simulink model "forme_canoniche"  (R2021b)
settings: Solver=ode3  StartTime=0.0  StopTime=2  FixedStep=Ts  RelTol=1e-3
values from neighbouring files (symbols this model uses):
  a = a(2:end)    [script.m]
  b = 2    [script.m]
  R = 1    [script.m]
settings Model: Creator=antony  LastModifiedBy=antony

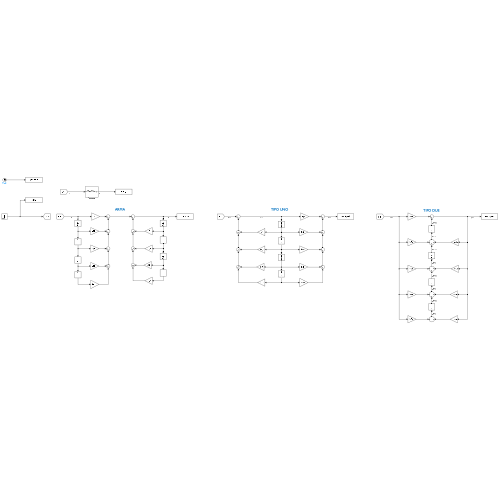
[thumbnail: Simulink's stored preview of the top-level diagram]
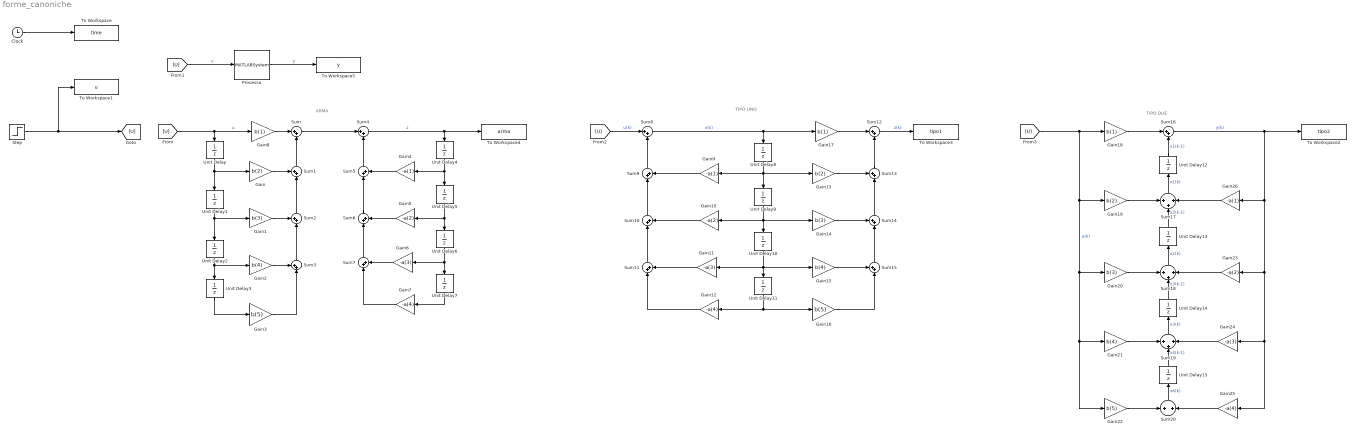
== system forme_canoniche ==
  note: ARMA
  note: TIPO UNO
  note: TIPO DUE
  Clock : Clock
  Gain : Gain  Gain=b(2)
  Gain1 : Gain  Gain=b(3)
  Gain10 : Gain  Gain=-a(2)
  Gain11 : Gain  Gain=-a(3)
  Gain12 : Gain  Gain=-a(4)
  Gain13 : Gain  Gain=b(2)
  Gain14 : Gain  Gain=b(3)
  Gain15 : Gain  Gain=b(4)
  Gain16 : Gain  Gain=b(5)
  Gain17 : Gain  Gain=b(1)
  Gain18 : Gain  Gain=b(1)
  Gain19 : Gain  Gain=b(2)
  Gain2 : Gain  Gain=b(4)
  Gain20 : Gain  Gain=b(3)
  Gain21 : Gain  Gain=b(4)
  Gain22 : Gain  Gain=b(5)
  Gain23 : Gain  Gain=-a(2)
  Gain24 : Gain  Gain=-a(3)
  Gain25 : Gain  Gain=-a(4)
  Gain26 : Gain  Gain=-a(1)
  Gain3 : Gain  Gain=b(5)
  Gain4 : Gain  Gain=-a(1)
  Gain5 : Gain  Gain=-a(2)
  Gain6 : Gain  Gain=-a(3)
  Gain7 : Gain  Gain=-a(4)
  Gain8 : Gain  Gain=b(1)
  Gain9 : Gain  Gain=-a(1)
  Processo : MATLABSystem  System=linSysObj  SimulateUsing=Interpreted execution
      mask Type: linSysObj
      mask Display:
      | disp('Black box');
      | port_label('input',1,'u');
      | port_label('output',1,'y');
  Step : Step  Time=0  After=R  SampleTime=0
  Sum{,4..12,16} (11 alike) : Sum  Inputs=|++
  Sum{1..3,13..15} (6 alike) : Sum  Inputs=++|
  Sum17 : Sum  Inputs=+|+|+
  Sum18 : Sum  Inputs=+|+|+
  Sum19 : Sum  Inputs=+|+|+
  Sum20 : Sum  Inputs=+|+
  To Workspace : ToWorkspace  VariableName=time  SampleTime=-1
      settings: Save2DSignal=2-D array (concatenate along first dimension)
  To Workspace1 : ToWorkspace  VariableName=u  SampleTime=-1
      settings: Save2DSignal=2-D array (concatenate along first dimension)
  To Workspace2 : ToWorkspace  VariableName=tipo2  SampleTime=-1
      settings: Save2DSignal=2-D array (concatenate along first dimension)
  To Workspace3 : ToWorkspace  VariableName=tipo1  SampleTime=-1
      settings: Save2DSignal=2-D array (concatenate along first dimension)
  To Workspace4 : ToWorkspace  VariableName=arma  SampleTime=-1
      settings: Save2DSignal=2-D array (concatenate along first dimension)
  To Workspace5 : ToWorkspace  VariableName=y  SampleTime=-1
      settings: Save2DSignal=2-D array (concatenate along first dimension)
  Unit Delay{,1..15} (16 alike) : UnitDelay  SampleTime=-1  HasFrameUpgradeWarning=on
  wires:
  Clock/1 -> To Workspace/1
  Step/1 -> To Workspace1/1, [U]
  [U] -> Gain8/1, Unit Delay/1  "u"
  Sum1/1 -> Sum/2
  Sum2/1 -> Sum1/2
  Sum3/1 -> Sum2/2
  Sum/1 -> Sum4/1
  Sum5/1 -> Sum4/2
  Sum6/1 -> Sum5/1
  Sum7/1 -> Sum6/1
  Unit Delay/1 -> Gain/1, Unit Delay1/1
  Unit Delay1/1 -> Unit Delay2/1, Gain1/1
  Unit Delay2/1 -> Unit Delay3/1, Gain2/1
  Unit Delay3/1 -> Gain3/1
  Gain3/1 -> Sum3/2
  Gain2/1 -> Sum3/1
  Gain1/1 -> Sum2/1
  Gain/1 -> Sum1/1
  Unit Delay4/1 -> Unit Delay5/1, Gain4/1
  Unit Delay5/1 -> Unit Delay6/1, Gain5/1
  Unit Delay6/1 -> Unit Delay7/1, Gain6/1
  Unit Delay7/1 -> Gain7/1
  Gain7/1 -> Sum7/1
  Gain6/1 -> Sum7/2
  Gain5/1 -> Sum6/2
  Gain4/1 -> Sum5/2
  Gain8/1 -> Sum/1
  Sum4/1 -> Unit Delay4/1, To Workspace4/1  "z"
  Unit Delay8/1 -> Gain13/1, Unit Delay9/1, Gain9/1
  Unit Delay11/1 -> Gain12/1, Gain16/1
  Unit Delay9/1 -> Gain14/1, Unit Delay10/1, Gain10/1
  Sum8/1 -> Unit Delay8/1, Gain17/1  "x(k)"
  [U] -> Sum8/1  "u(k)"
  Gain17/1 -> Sum12/1
  Sum13/1 -> Sum12/2
  Sum15/1 -> Sum14/2
  Unit Delay10/1 -> Gain11/1, Unit Delay11/1, Gain15/1
  Gain14/1 -> Sum14/1
  Sum14/1 -> Sum13/2
  Gain15/1 -> Sum15/1
  Gain13/1 -> Sum13/1
  Gain16/1 -> Sum15/2
  Sum9/1 -> Sum8/2
  Gain9/1 -> Sum9/2
  Sum10/1 -> Sum9/1
  Gain10/1 -> Sum10/2
  Sum11/1 -> Sum10/1
  Gain11/1 -> Sum11/2
  Gain12/1 -> Sum11/1
  Gain18/1 -> Sum16/1
  Unit Delay12/1 -> Sum16/2  "x1(k-1)"
  Sum17/1 -> Unit Delay12/1  "x1(k)"
  Unit Delay13/1 -> Sum17/2  "x2(k-1)"
  Unit Delay14/1 -> Sum18/2  "x3(k-1)"
  Sum18/1 -> Unit Delay13/1  "x2(k)"
  Sum19/1 -> Unit Delay14/1  "x3(k)"
  Unit Delay15/1 -> Sum19/2  "x4(k-1)"
  Sum20/1 -> Unit Delay15/1  "x4(k)"
  Gain25/1 -> Sum20/2
  Gain22/1 -> Sum20/1
  [U] -> Gain21/1, Gain22/1, Gain20/1, Gain19/1, Gain18/1  "u(k)"
  Sum16/1 -> To Workspace2/1, Gain25/1, Gain24/1, Gain23/1, Gain26/1  "y(k)"
  Gain26/1 -> Sum17/3
  Gain21/1 -> Sum19/1
  Gain19/1 -> Sum17/1
  Gain20/1 -> Sum18/1
  Gain23/1 -> Sum18/3
  Gain24/1 -> Sum19/3
  Sum12/1 -> To Workspace3/1  "z(k)"
  [U] -> Processo/1  "u"
  Processo/1 -> To Workspace5/1  "y"
